simulink model "MPC_point_4"  (R2022a)
settings: Solver=VariableStepAuto  StartTime=0.0  StopTime=20  RelTol=1e-3
values from neighbouring files (symbols this model uses):
  C = [0       1      0  0 ... (first row only)    [main.m]
  C_states = eye(length(A))    [main.m]
  D_states = zeros(length(B), 1)    [main.m]
  N4 = 5    [main.m]
  N5 = 100    [main.m]
  N6 = 100    [main.m]
  N7 = 100    [main.m]
  Q4 = Q_d    [main.m]
  Q5 = Q_d    [main.m]
  Q6 = 50 * Q_d    [main.m]
  Q7 = Q_d    [main.m]
  R4 = R_d    (= 10000)    [main.m]
  R5 = R_d    (= 10000)    [main.m]
  R6 = R_d    (= 10000)    [main.m]
  R7 = 50 * R_d    (= 500000)    [main.m]
  S4 = P_d    [main.m]
  S5 = P_d    [main.m]
  S6 = P_d    [main.m]
  S7 = P_d    [main.m]
  sysd = c2d(sys,T_sampling)    [main.m]
  T_sampling = 2*pi/omega_sampling    [main.m]
  u_max = deg2rad(15)    [main.m]
  u_min = deg2rad(-15)    [main.m]
  x0 = [deg2rad(0) deg2rad(15) 0 -300]    [main.m]
  x_ref = [0 0 0 0]    [main.m]
undefined symbols (not defined in the file or in its folder): Klqr_d, mpc_point_3
settings Model: Creator=PaoloA  LastModifiedBy=g_mor
settings DebuggingCC: UnconnectedInputMsg=warning  UnconnectedOutputMsg=warning  UnconnectedLineMsg=warning
settings RTWCC: DLArmComputeVersion=19.05

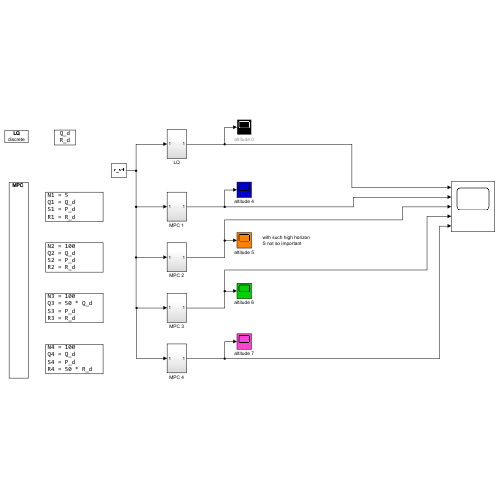
[thumbnail: Simulink's stored preview of the top-level diagram]
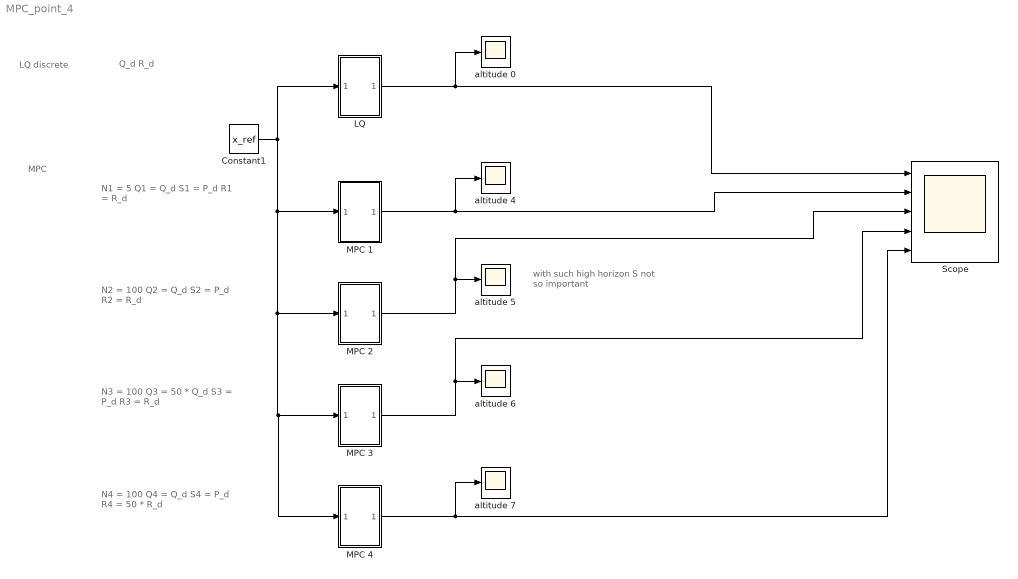
== system MPC_point_4 ==
  note: with such high horizon
      | S not so important
  note: N1 = 5
      | Q1 = Q_d
      | S1 = P_d
      | R1 = R_d
  note: LQ
      | discrete
  note: MPC
  note: Q_d
      | R_d
  note: N2 = 100
      | Q2 = Q_d
      | S2 = P_d
      | R2 = R_d
  note: N3 = 100
      | Q3 = 50 * Q_d
      | S3 = P_d
      | R3 = R_d
  note: N4 = 100
      | Q4 = Q_d
      | S4 = P_d
      | R4 = 50 * R_d
  Constant1 : Constant  Value=x_ref
  LQ : Subsystem
  MPC 1 : Subsystem
  MPC 2 : Subsystem
  MPC 3 : Subsystem
  MPC 4 : Subsystem
  Scope : Scope  NumInputPorts=5
  altitude {0,4..7} (5 alike) : Scope
  wires:
  MPC 1/1(Out1) -> Scope/2, altitude 4/1
  LQ/1(Out1) -> Scope/1, altitude 0/1
  MPC 2/1(Out1) -> Scope/3, altitude 5/1
  MPC 3/1(Out1) -> Scope/4, altitude 6/1
  MPC 4/1(Out1) -> Scope/5, altitude 7/1
  Constant1/1 -> LQ/1(In1), MPC 4/1(In1), MPC 3/1(In1), MPC 2/1(In1), MPC 1/1(In1)

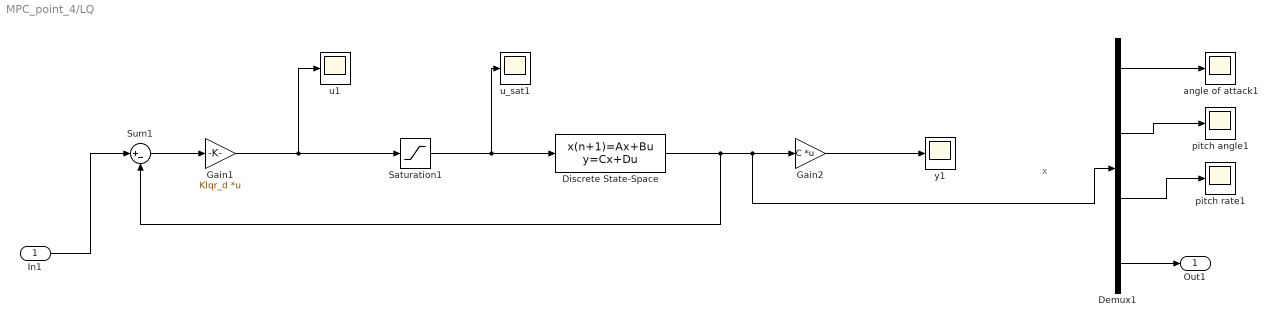
== system MPC_point_4/LQ ==
  note: x
  In1 : Inport
  Demux1 : Demux
  Discrete State-Space : DiscreteStateSpace  A=sysd.A  B=sysd.B  C=C_states  D=D_states  InitialCondition=x0  SampleTime=T_sampling
  Gain1 : Gain  Gain=Klqr_d  Multiplication=Matrix(K*u)
  Gain2 : Gain  Gain=C  Multiplication=Matrix(K*u)
  Saturation1 : Saturate  UpperLimit=u_max  LowerLimit=u_min
  Sum1 : Sum  Inputs=|+-
  angle of attack1 : Scope
  pitch angle1 : Scope
  pitch rate1 : Scope
  u1 : Scope
  u_sat1 : Scope
  y1 : Scope
  Out1 : Outport
  wires:
  Gain2/1 -> y1/1
  Discrete State-Space/1 -> Demux1/1, Gain2/1, Sum1/2
  Saturation1/1 -> Discrete State-Space/1, u_sat1/1
  Gain1/1 -> u1/1, Saturation1/1
  Demux1/4 -> Out1/1
  Demux1/1 -> angle of attack1/1
  Sum1/1 -> Gain1/1
  Demux1/2 -> pitch angle1/1
  Demux1/3 -> pitch rate1/1
  In1/1 -> Sum1/1

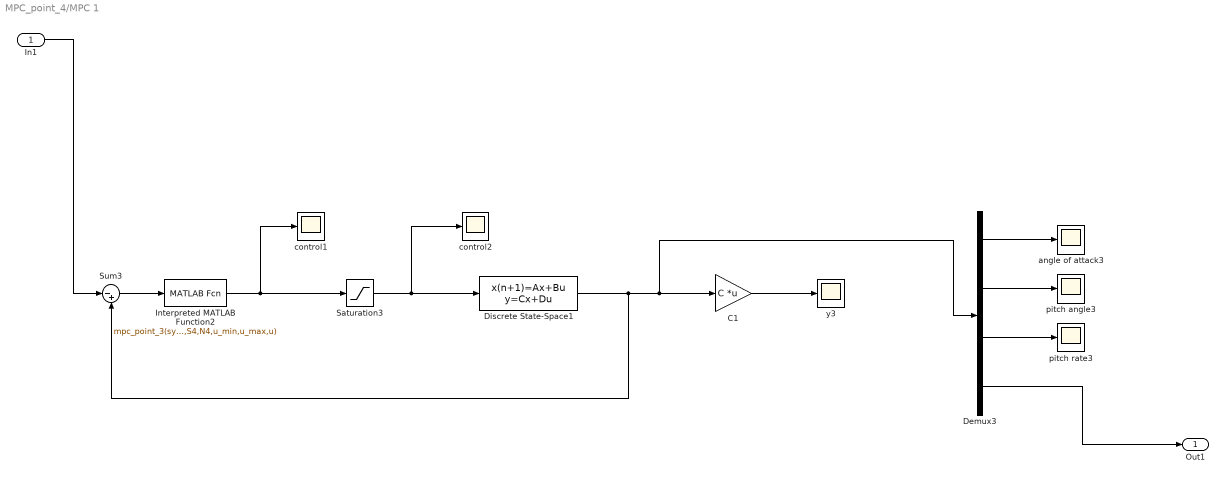
== system MPC_point_4/MPC 1 ==
  In1 : Inport
  C1 : Gain  Gain=C  Multiplication=Matrix(K*u)
  Demux3 : Demux
  Discrete State-Space1 : DiscreteStateSpace  A=sysd.A  B=sysd.B  C=C_states  D=D_states  InitialCondition=x0  SampleTime=T_sampling
  Interpreted MATLAB Function2 : MATLABFcn  MATLABFcn=mpc_point_3(sysd.A,sysd.B,Q4,R4,S4,N4,u_min,u_max,u)  OutputDimensions=1
  Saturation3 : Saturate  UpperLimit=u_max  LowerLimit=u_min
  Sum3 : Sum  Inputs=|-+
  angle of attack3 : Scope
  control1 : Scope
  control2 : Scope
  pitch angle3 : Scope
  pitch rate3 : Scope
  y3 : Scope
  Out1 : Outport
  wires:
  Demux3/1 -> angle of attack3/1
  Saturation3/1 -> Discrete State-Space1/1, control2/1
  Demux3/3 -> pitch rate3/1
  Discrete State-Space1/1 -> C1/1, Demux3/1, Sum3/2
  Demux3/2 -> pitch angle3/1
  C1/1 -> y3/1
  Interpreted MATLAB Function2/1 -> Saturation3/1, control1/1
  Sum3/1 -> Interpreted MATLAB Function2/1
  Demux3/4 -> Out1/1
  In1/1 -> Sum3/1

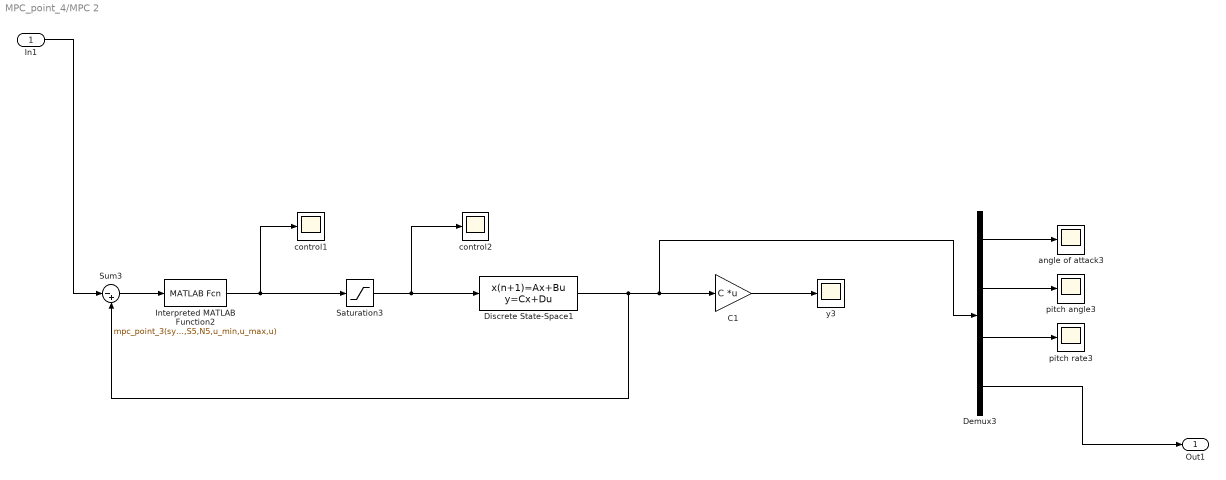
== system MPC_point_4/MPC 2 ==
  In1 : Inport
  C1 : Gain  Gain=C  Multiplication=Matrix(K*u)
  Demux3 : Demux
  Discrete State-Space1 : DiscreteStateSpace  A=sysd.A  B=sysd.B  C=C_states  D=D_states  InitialCondition=x0  SampleTime=T_sampling
  Interpreted MATLAB Function2 : MATLABFcn  MATLABFcn=mpc_point_3(sysd.A,sysd.B,Q5,R5,S5,N5,u_min,u_max,u)  OutputDimensions=1
  Saturation3 : Saturate  UpperLimit=u_max  LowerLimit=u_min
  Sum3 : Sum  Inputs=|-+
  angle of attack3 : Scope
  control1 : Scope
  control2 : Scope
  pitch angle3 : Scope
  pitch rate3 : Scope
  y3 : Scope
  Out1 : Outport
  wires:
  Demux3/1 -> angle of attack3/1
  Saturation3/1 -> Discrete State-Space1/1, control2/1
  Demux3/3 -> pitch rate3/1
  Discrete State-Space1/1 -> C1/1, Demux3/1, Sum3/2
  Demux3/2 -> pitch angle3/1
  C1/1 -> y3/1
  Interpreted MATLAB Function2/1 -> Saturation3/1, control1/1
  Sum3/1 -> Interpreted MATLAB Function2/1
  Demux3/4 -> Out1/1
  In1/1 -> Sum3/1

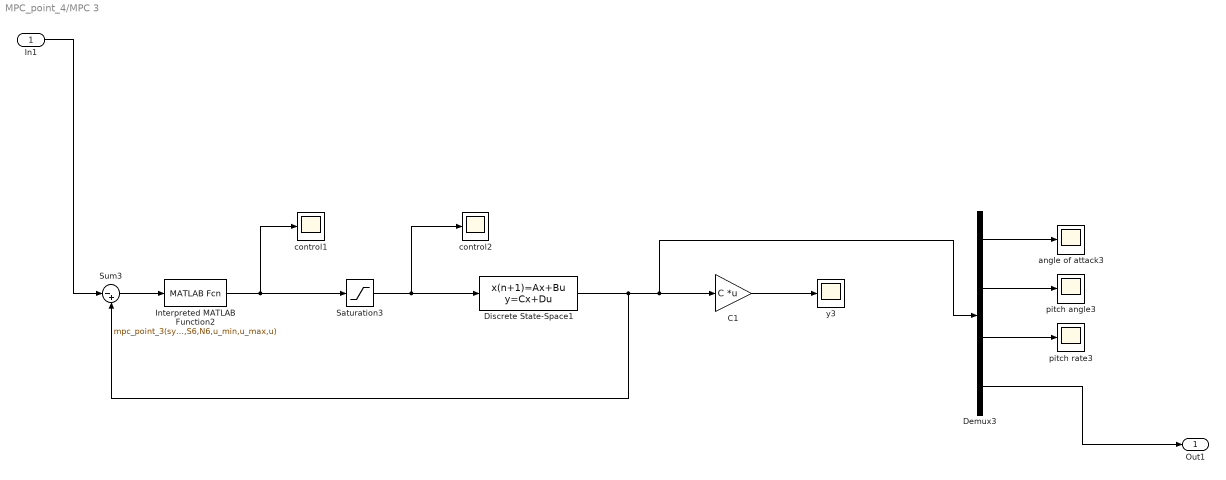
== system MPC_point_4/MPC 3 ==
  In1 : Inport
  C1 : Gain  Gain=C  Multiplication=Matrix(K*u)
  Demux3 : Demux
  Discrete State-Space1 : DiscreteStateSpace  A=sysd.A  B=sysd.B  C=C_states  D=D_states  InitialCondition=x0  SampleTime=T_sampling
  Interpreted MATLAB Function2 : MATLABFcn  MATLABFcn=mpc_point_3(sysd.A,sysd.B,Q6,R6,S6,N6,u_min,u_max,u)  OutputDimensions=1
  Saturation3 : Saturate  UpperLimit=u_max  LowerLimit=u_min
  Sum3 : Sum  Inputs=|-+
  angle of attack3 : Scope
  control1 : Scope
  control2 : Scope
  pitch angle3 : Scope
  pitch rate3 : Scope
  y3 : Scope
  Out1 : Outport
  wires:
  Demux3/1 -> angle of attack3/1
  Saturation3/1 -> Discrete State-Space1/1, control2/1
  Demux3/3 -> pitch rate3/1
  Discrete State-Space1/1 -> C1/1, Demux3/1, Sum3/2
  Demux3/2 -> pitch angle3/1
  C1/1 -> y3/1
  Interpreted MATLAB Function2/1 -> Saturation3/1, control1/1
  Sum3/1 -> Interpreted MATLAB Function2/1
  Demux3/4 -> Out1/1
  In1/1 -> Sum3/1

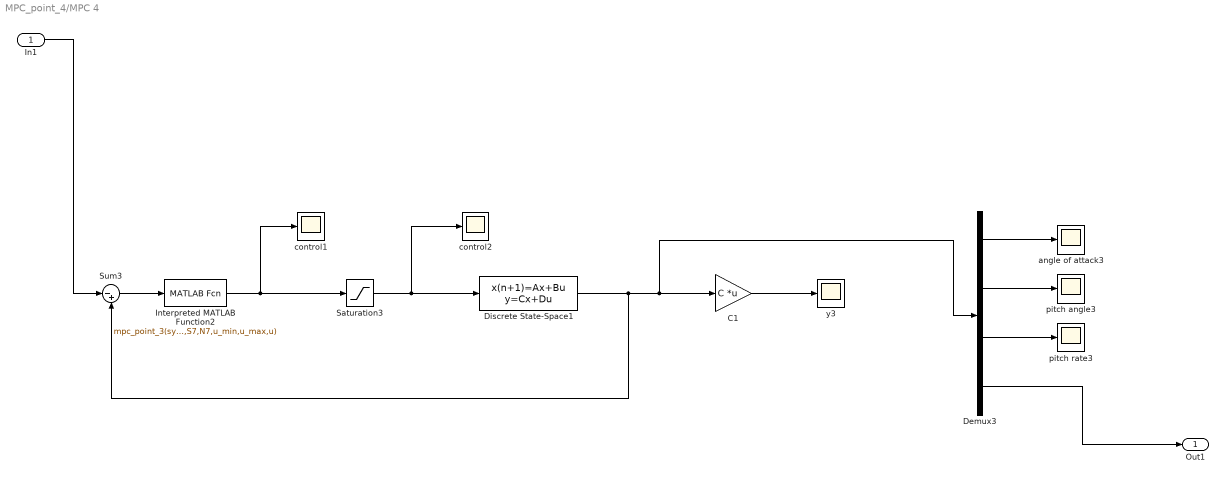
== system MPC_point_4/MPC 4 ==
  In1 : Inport
  C1 : Gain  Gain=C  Multiplication=Matrix(K*u)
  Demux3 : Demux
  Discrete State-Space1 : DiscreteStateSpace  A=sysd.A  B=sysd.B  C=C_states  D=D_states  InitialCondition=x0  SampleTime=T_sampling
  Interpreted MATLAB Function2 : MATLABFcn  MATLABFcn=mpc_point_3(sysd.A,sysd.B,Q7,R7,S7,N7,u_min,u_max,u)  OutputDimensions=1
  Saturation3 : Saturate  UpperLimit=u_max  LowerLimit=u_min
  Sum3 : Sum  Inputs=|-+
  angle of attack3 : Scope
  control1 : Scope
  control2 : Scope
  pitch angle3 : Scope
  pitch rate3 : Scope
  y3 : Scope
  Out1 : Outport
  wires:
  Demux3/1 -> angle of attack3/1
  Saturation3/1 -> Discrete State-Space1/1, control2/1
  Demux3/3 -> pitch rate3/1
  Discrete State-Space1/1 -> C1/1, Demux3/1, Sum3/2
  Demux3/2 -> pitch angle3/1
  C1/1 -> y3/1
  Interpreted MATLAB Function2/1 -> Saturation3/1, control1/1
  Sum3/1 -> Interpreted MATLAB Function2/1
  Demux3/4 -> Out1/1
  In1/1 -> Sum3/1
